simulink model "ABS1"  (R2018a)
settings: Solver=VariableStepAuto  StartTime=0.0  StopTime=5  RelTol=1e-3
settings Model: Creator=Administrator  LastModifiedBy=Yorke
settings CodeAppCC: StateflowObjectComments=on

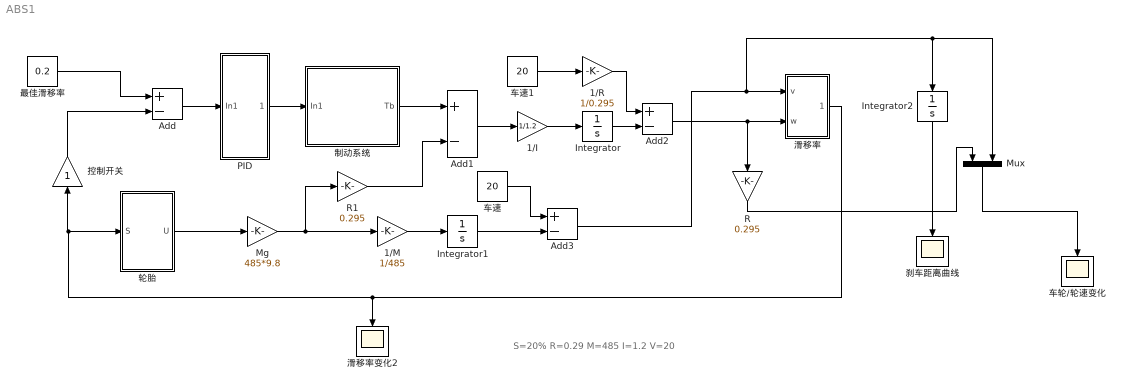
== system ABS1 ==
  note: S=20%
      | R=0.29
      | M=485
      | I=1.2
      | V=20
  1/I : Gain  Gain=1/1.2
  1/M : Gain  Gain=1/485
  1/R : Gain  Gain=1/0.295
  Add{,1..3} (4 alike) : Sum  Inputs=+-
  Integrator : Integrator  LimitOutput=on  UpperSaturationLimit=1000  LowerSaturationLimit=-1000
  Integrator1 : Integrator  LimitOutput=on  UpperSaturationLimit=1000  LowerSaturationLimit=-1000
  Integrator2 : Integrator
  Mg : Gain  Gain=485*9.8
  Mux : Mux  Inputs=2
  PID : Subsystem
  "R " : Gain  Gain=0.295
  R1 : Gain  Gain=0.295
  制动系统 : Subsystem
  刹车距离曲线 : Scope
  控制开关 : Gain
  "最佳滑移率 " : Constant  Value=0.2
  滑移率 : Subsystem
  滑移率变化2 : Scope
  "车轮/轮速变化 " : Scope
  车速 : Constant  Value=20
  车速1 : Constant  Value=20
  轮胎 : Subsystem
  wires:
  "最佳滑移率 "/1 -> Add/1
  Add/1 -> PID/1(In1)
  PID/1(Out1) -> 制动系统/1(In1)
  制动系统/1("Tb ") -> Add1/1
  Add1/1 -> 1/I/1
  车速1/1 -> 1/R/1
  1/I/1 -> Integrator/1
  Integrator/1 -> Add2/2
  1/R/1 -> Add2/1
  Add2/1 -> "R "/1, 滑移率/2(w)
  轮胎/1("U ") -> Mg/1
  Mg/1 -> R1/1, 1/M/1
  R1/1 -> Add1/2
  1/M/1 -> Integrator1/1
  Integrator1/1 -> Add3/2
  车速/1 -> Add3/1
  Add3/1 -> Integrator2/1, Mux/2, 滑移率/1(v)
  Integrator2/1 -> 刹车距离曲线/1
  Mux/1 -> "车轮/轮速变化 "/1
  "R "/1 -> Mux/1
  滑移率/1(Out2) -> 滑移率变化2/1, 轮胎/1(S), 控制开关/1
  控制开关/1 -> Add/2

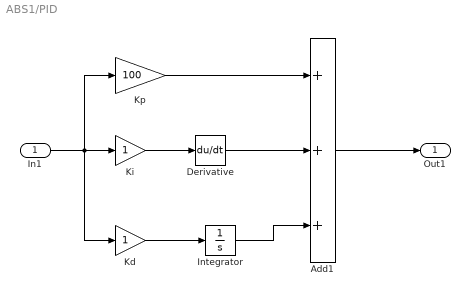
== system ABS1/PID ==
  In1 : Inport
  Add1 : Sum  Inputs=+++
  Derivative : Derivative
  Integrator : Integrator
  Kd : Gain
  Ki : Gain
  "Kp " : Gain  Gain=100
  Out1 : Outport
  wires:
  Integrator/1 -> Add1/3
  Kd/1 -> Integrator/1
  In1/1 -> "Kp "/1, Kd/1, Ki/1
  Derivative/1 -> Add1/2
  "Kp "/1 -> Add1/1
  Add1/1 -> Out1/1
  Ki/1 -> Derivative/1

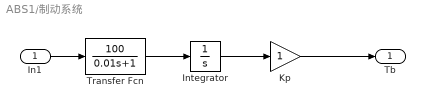
== system ABS1/制动系统 ==
  In1 : Inport
  Integrator : Integrator
  Kp : Gain
  Transfer Fcn : TransferFcn  Numerator=[100]  Denominator=[0.01 1]
  "Tb " : Outport
  wires:
  Transfer Fcn/1 -> Integrator/1
  Kp/1 -> "Tb "/1
  Integrator/1 -> Kp/1
  In1/1 -> Transfer Fcn/1

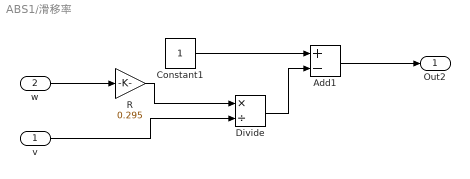
== system ABS1/滑移率 ==
  v : Inport
  w : Inport  Port=2
  Add1 : Sum  Inputs=+-
  Constant1 : Constant
  Divide : Product  Inputs=*/
  R : Gain  Gain=0.295
  Out2 : Outport
  wires:
  w/1 -> R/1
  Add1/1 -> Out2/1
  v/1 -> Divide/2
  Divide/1 -> Add1/2
  R/1 -> Divide/1
  Constant1/1 -> Add1/1

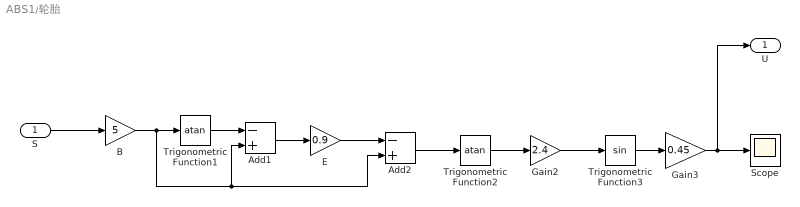
== system ABS1/轮胎 ==
  S : Inport
  Add1 : Sum  Inputs=-+
  Add2 : Sum  Inputs=-+
  B : Gain  Gain=5
  E : Gain  Gain=0.9
  Gain2 : Gain  Gain=2.4
  Gain3 : Gain  Gain=0.45
  Scope : Scope
  Trigonometric Function1 : Trigonometry  Operator=atan
  Trigonometric Function2 : Trigonometry  Operator=atan
  Trigonometric Function3 : Trigonometry
  "U " : Outport
  wires:
  Add2/1 -> Trigonometric Function2/1
  Trigonometric Function2/1 -> Gain2/1
  Trigonometric Function1/1 -> Add1/1
  Add1/1 -> E/1
  B/1 -> Add1/2, Add2/2, Trigonometric Function1/1
  S/1 -> B/1
  E/1 -> Add2/1
  Gain3/1 -> "U "/1, Scope/1
  Gain2/1 -> Trigonometric Function3/1
  Trigonometric Function3/1 -> Gain3/1
